simulink model "Assignment1"  (R2024a)
settings: Solver=FixedStepAuto  StartTime=0.0  StopTime=30  FixedStep=1e-3  RelTol=1e-3  EnableMultiTasking=on
undefined symbols (not defined in the file): D0, D1, D10, D11, D12, D13, D2, D3, D4, D5, D6, D7, D8, D9, PTA0, PTA1, PTA2, PTB23, PTB9, PTC16, PTC17, PTC2, PTC3, PTC4, PTD0, PTD1, PTD2, PTD3
libraries: frdmk64flib x19, dspstat3 x1
settings Model: ExtModeTrigDuration=5  Creator=raymo  LastModifiedBy=peter
settings SolverCC: AlgebraicLoopSolver=TrustRegion
settings OptimizationCC: EnhancedBackFolding=on  PassReuseOutputArgsAs=Individual arguments  ZeroExternalMemoryAtStartup=off  ZeroInternalMemoryAtStartup=off  MaxStackSize=64  OptimizeBlockOrder=speed  DifferentSizesBufferReuse=on  OptimizationCustomize=off  EfficientTunableParamExpr=on
settings DebuggingCC: ParameterTunabilityLossMsg=error  UnconnectedInputMsg=warning  UnconnectedOutputMsg=warning  UnconnectedLineMsg=warning
settings HardwareCC: ProdBitPerPointer=32  ProdBitPerSizeT=32  ProdBitPerPtrDiffT=32  ProdLargestAtomicInteger=Long  ProdLargestAtomicFloat=Double  ProdWordSize=32  ProdHWDeviceType=ARM Compatible->ARM Cortex
settings ModelReferenceCC: EnableRefExpFcnMdlSchedulingChecks=on
settings SFSimCC: MATLABDynamicMemAlloc=off
settings RTWCC: Description=Embedded Coder  SystemTargetFile=ert.tlc  HardwareBoard=NXP FRDM-K64F  TLCOptions="-aInlineSetEventsForThisBaseRateFcn=TLC_FALSE -aSuppressMultiTaskScheduler=TLC_FALSE  -aRateBasedStepFcn=0"  TemplateMakefile=ert_default_tmf  Toolchain=GNU Tools for ARM Embedded Processors  GPUComputeCapability=3.5
settings CodeAppCC: ForceParamTrailComments=on  IgnoreCustomStorageClasses=off  OperatorAnnotations=on  SimulinkDataObjDesc=on  SFDataObjDesc=on  InsertBlockDesc=on

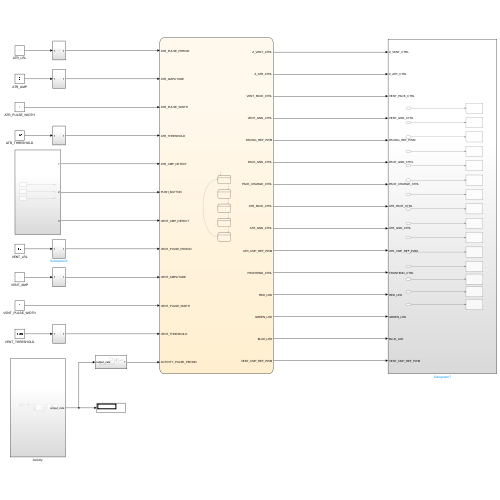
[thumbnail: Simulink's stored preview of the top-level diagram]
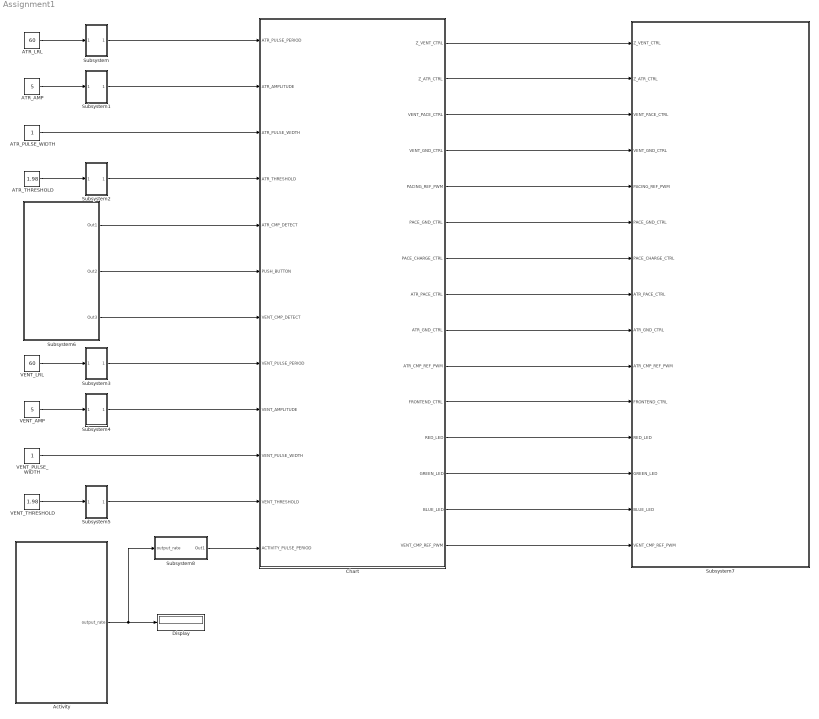
== system Assignment1 ==
  ATR_AMP : Constant  Value=5
  ATR_LRL : Constant  Value=60
  ATR_PULSE_WIDTH : Constant
  ATR_THRESHOLD : Constant  Value=1.98
  Activity : Subsystem
  Chart : Stateflow chart  TreatAsAtomicUnit=on
      settings: PortSchema="{\"entries\":[{\"content\":{\"sides\":[{\"content\":{\"connectorIds\":[\"In1\",\"In2\",\"In3\",\"In4\",\"In5\",\"In6\",\"In9\",\"In7\",\"In8\",\"In10\",\"In11\",\"In12\"]},\"type\":\"ConnectorPlacement.EquallySpacedRectSide\",\"uuid\":\"1d074b9c-7cc8-4198-85a6-5618993573f0\"},{\"content\":{\"connectorIds\":[\"Out1\",\"Out2\",\"Out3\",\"Out4\",\"Out5\",\"Out6\",\"Out7\",\"Out8\",\"Out9\",\"Out10\",\"Out11\",\"Out12\",\"Out13\",\"Out14\",\"Out15\"],\"side\":\"RIGHT\"},\"type\":\"ConnectorPlacement.EquallySpacedRectSide\",\"uuid\":\"14c2042e-8be8-4cb1-bcfb-7c1019a33e21\"},{\"content\":{\"side\":\"TOP\"},\"type\":\"ConnectorPlacement.EquallySpacedRectSide\",\"uuid\":\"e4fcd7b9-cecf-490a-a51f-afb907c3ace7\"}]},\"type\":\"ConnectorPlacement.EquallySpacedConnector\",\"uuid\":\"e4f7c1e4-ab35-4f24-879f-75d9e4e0e882\"}],\"packageUris\":[\"http://schema.mathworks.com/mf0/Connector/R2020b\"],\"version\":\"1.0\"}"
  Display : Display
  Subsystem : Subsystem
  Subsystem1 : Subsystem
  Subsystem2 : Subsystem
  Subsystem3 : Subsystem
  Subsystem4 : Subsystem
  Subsystem5 : Subsystem
  Subsystem6 : Subsystem
  Subsystem7 : Subsystem
  Subsystem8 : Subsystem
  VENT_AMP : Constant  Value=5
  VENT_LRL : Constant  Value=60
  VENT_PULSE_WIDTH : Constant
  VENT_THRESHOLD : Constant  Value=1.98
  wires:
  ATR_PULSE_WIDTH/1 -> Chart/3(ATR_PULSE_WIDTH)
  ATR_LRL/1 -> Subsystem/1(In1)
  Subsystem/1(Out1) -> Chart/1(ATR_PULSE_PERIOD)
  ATR_AMP/1 -> Subsystem1/1(In1)
  Subsystem1/1(Out1) -> Chart/2(ATR_AMPLITUDE)
  ATR_THRESHOLD/1 -> Subsystem2/1(In1)
  Subsystem2/1(Out1) -> Chart/4(ATR_THRESHOLD)
  Subsystem3/1(Out1) -> Chart/7(VENT_PULSE_PERIOD)
  VENT_LRL/1 -> Subsystem3/1(In1)
  VENT_AMP/1 -> Subsystem4/1(In1)
  Subsystem4/1(Out1) -> Chart/8(VENT_AMPLITUDE)
  VENT_PULSE_WIDTH/1 -> Chart/10(VENT_PULSE_WIDTH)
  VENT_THRESHOLD/1 -> Subsystem5/1(In1)
  Subsystem5/1(Out1) -> Chart/11(VENT_THRESHOLD)
  Subsystem6/1(Out1) -> Chart/5(ATR_CMP_DETECT)
  Subsystem6/2(Out2) -> Chart/6(PUSH_BUTTON)
  Subsystem6/3(Out3) -> Chart/9(VENT_CMP_DETECT)
  Chart/1(Z_VENT_CTRL) -> Subsystem7/1(Z_VENT_CTRL)
  Chart/2(Z_ATR_CTRL) -> Subsystem7/2(Z_ATR_CTRL)
  Chart/3(VENT_PACE_CTRL) -> Subsystem7/3(VENT_PACE_CTRL)
  Chart/4(VENT_GND_CTRL) -> Subsystem7/4(VENT_GND_CTRL)
  Chart/5(PACING_REF_PWM) -> Subsystem7/5(PACING_REF_PWM)
  Chart/6(PACE_GND_CTRL) -> Subsystem7/6(PACE_GND_CTRL)
  Chart/7(PACE_CHARGE_CTRL) -> Subsystem7/7(PACE_CHARGE_CTRL)
  Chart/8(ATR_PACE_CTRL) -> Subsystem7/8(ATR_PACE_CTRL)
  Chart/9(ATR_GND_CTRL) -> Subsystem7/9(ATR_GND_CTRL)
  Chart/10(ATR_CMP_REF_PWM) -> Subsystem7/10(ATR_CMP_REF_PWM)
  Chart/11(FRONTEND_CTRL) -> Subsystem7/11(FRONTEND_CTRL)
  Chart/12(RED_LED) -> Subsystem7/12(RED_LED)
  Chart/13(GREEN_LED) -> Subsystem7/13(GREEN_LED)
  Chart/15(VENT_CMP_REF_PWM) -> Subsystem7/15(VENT_CMP_REF_PWM)
  Activity/1(output_rate) -> Display/1, Subsystem8/1(output_rate)
  Subsystem8/1(Out1) -> Chart/12(ACTIVITY_PULSE_PERIOD)
  Chart/14(BLUE_LED) -> Subsystem7/14(BLUE_LED)

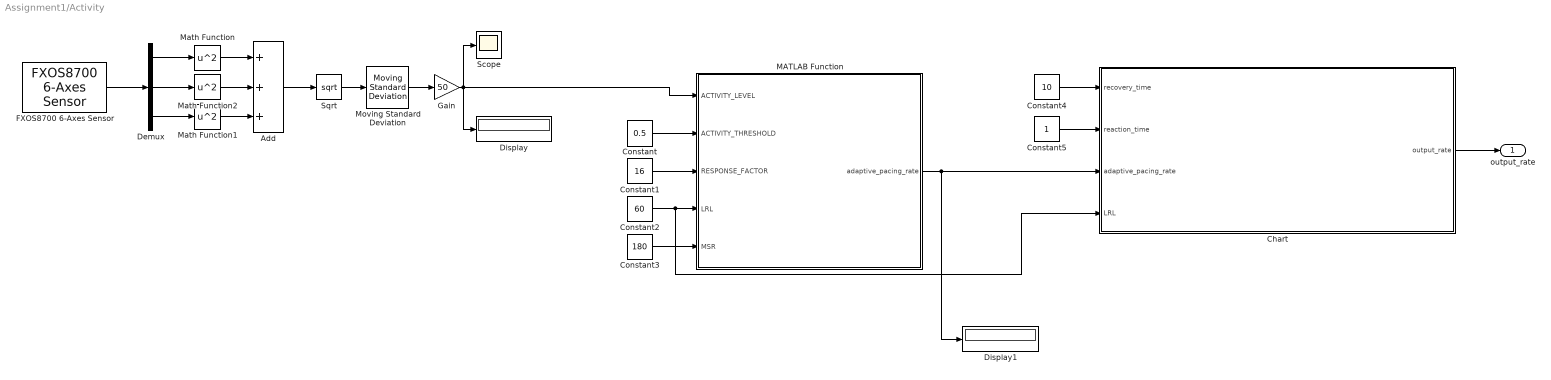
== system Assignment1/Activity ==
  Add : Sum  Inputs=+++
  Chart : Stateflow chart  TreatAsAtomicUnit=on
  Constant : Constant  Value=0.5
  Constant1 : Constant  Value=16
  Constant2 : Constant  Value=60
  Constant3 : Constant  Value=180
  Constant4 : Constant  Value=10
  Constant5 : Constant
  Demux : Demux  Outputs=3
  Display : Display
  Display1 : Display
  FXOS8700 6-Axes Sensor : frdmk64flib/FXOS8700 6-Axes Sensor  Activesensor=Accelerometer only  ODR=800Hz  HybridODR=400Hz  Accelfullrange=-4g to +4g  SampleTime=-1
  Gain : Gain  Gain=50
  MATLAB Function : MATLAB Function  TreatAsAtomicUnit=on
  Math Function : Math  Operator=square
  Math Function1 : Math  Operator=square
  Math Function2 : Math  Operator=square
  Moving Standard Deviation : dspstat3/Moving Standard Deviation  Method=Sliding window  ForgettingFactorPort=off  SpecifyWindowLength=on  WindowLength=4  OverlapLength=3  AllowArbitraryInputLength=off  ForgettingFactor=0.9  SimulateUsing=Interpreted execution
  Scope : Scope
  Sqrt : Sqrt
  output_rate : Outport
  wires:
  FXOS8700 6-Axes Sensor/1 -> Demux/1
  Demux/3 -> Math Function1/1
  Demux/2 -> Math Function2/1
  Demux/1 -> Math Function/1
  Math Function/1 -> Add/1
  Math Function2/1 -> Add/2
  Math Function1/1 -> Add/3
  Add/1 -> Sqrt/1
  Sqrt/1 -> Moving Standard Deviation/1
  Moving Standard Deviation/1 -> Gain/1
  Gain/1 -> Display/1, MATLAB Function/1(ACTIVITY_LEVEL), Scope/1
  Constant/1 -> MATLAB Function/2(ACTIVITY_THRESHOLD)
  Constant1/1 -> MATLAB Function/3(RESPONSE_FACTOR)
  Constant2/1 -> Chart/4(LRL), MATLAB Function/4(LRL)
  Constant3/1 -> MATLAB Function/5(MSR)
  MATLAB Function/1(adaptive_pacing_rate) -> Display1/1, Chart/3(adaptive_pacing_rate)
  Constant4/1 -> Chart/1(recovery_time)
  Constant5/1 -> Chart/2(reaction_time)
  Chart/1(output_rate) -> output_rate/1

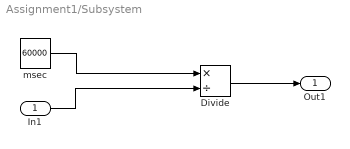
== system Assignment1/Subsystem ==
  In1 : Inport
  Divide : Product  Inputs=*/
  msec : Constant  Value=60000
  Out1 : Outport
  wires:
  Divide/1 -> Out1/1
  msec/1 -> Divide/1
  In1/1 -> Divide/2

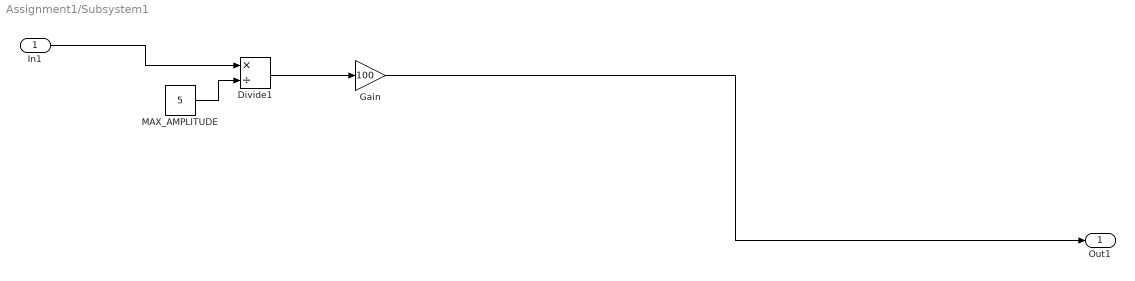
== system Assignment1/Subsystem1 ==
  In1 : Inport
  Divide1 : Product  Inputs=*/
  Gain : Gain  Gain=100
  MAX_AMPLITUDE : Constant  Value=5
  Out1 : Outport
  wires:
  Gain/1 -> Out1/1
  MAX_AMPLITUDE/1 -> Divide1/2
  In1/1 -> Divide1/1
  Divide1/1 -> Gain/1

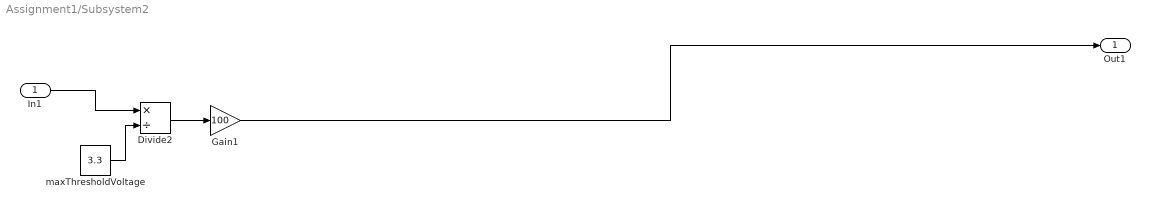
== system Assignment1/Subsystem2 ==
  In1 : Inport
  Divide2 : Product  Inputs=*/
  Gain1 : Gain  Gain=100
  maxThresholdVoltage : Constant  Value=3.3
  Out1 : Outport
  wires:
  Divide2/1 -> Gain1/1
  maxThresholdVoltage/1 -> Divide2/2
  In1/1 -> Divide2/1
  Gain1/1 -> Out1/1

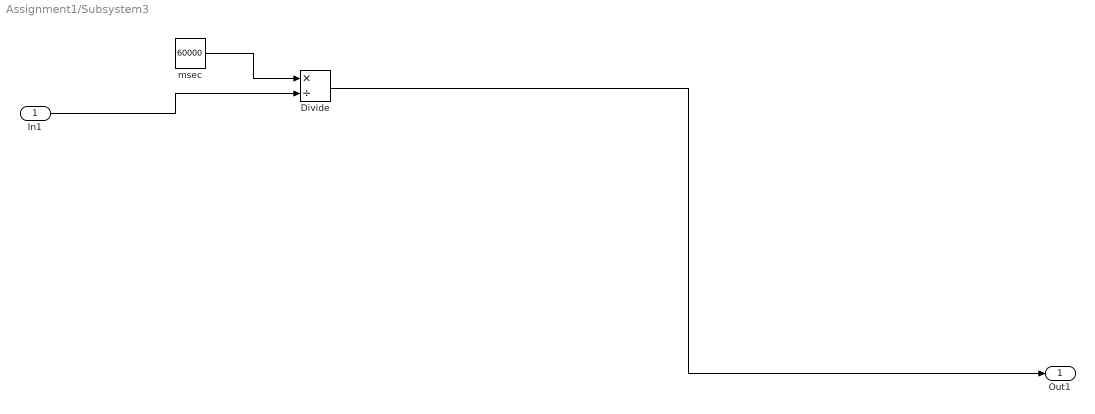
== system Assignment1/Subsystem3 ==
  In1 : Inport
  Divide : Product  Inputs=*/
  msec : Constant  Value=60000
  Out1 : Outport
  wires:
  Divide/1 -> Out1/1
  msec/1 -> Divide/1
  In1/1 -> Divide/2

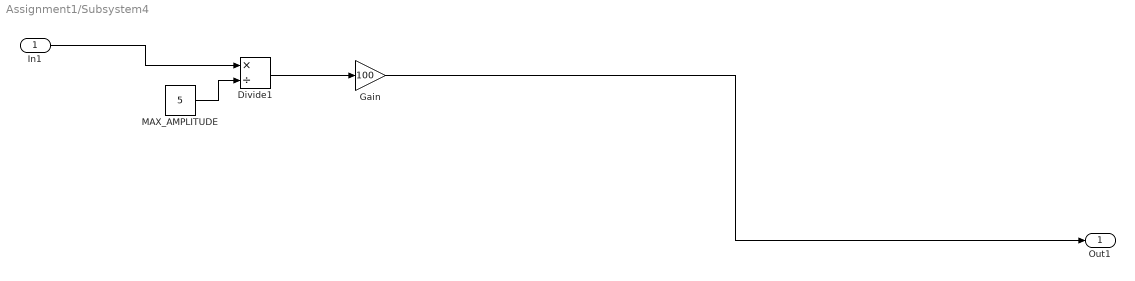
== system Assignment1/Subsystem4 ==
  In1 : Inport
  Divide1 : Product  Inputs=*/
  Gain : Gain  Gain=100
  MAX_AMPLITUDE : Constant  Value=5
  Out1 : Outport
  wires:
  Gain/1 -> Out1/1
  MAX_AMPLITUDE/1 -> Divide1/2
  In1/1 -> Divide1/1
  Divide1/1 -> Gain/1

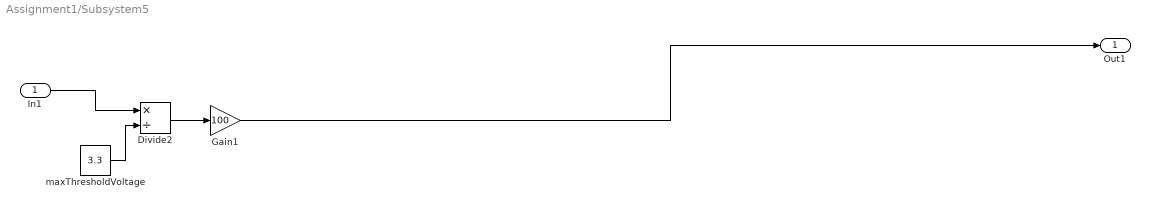
== system Assignment1/Subsystem5 ==
  In1 : Inport
  Divide2 : Product  Inputs=*/
  Gain1 : Gain  Gain=100
  maxThresholdVoltage : Constant  Value=3.3
  Out1 : Outport
  wires:
  Divide2/1 -> Gain1/1
  maxThresholdVoltage/1 -> Divide2/2
  In1/1 -> Divide2/1
  Gain1/1 -> Out1/1

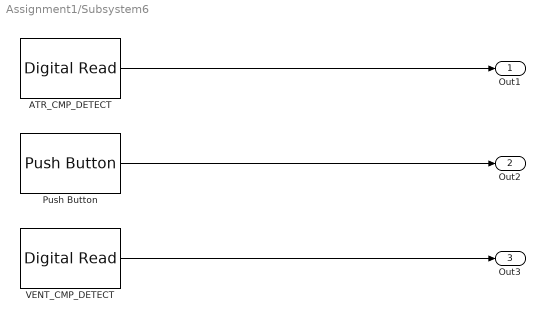
== system Assignment1/Subsystem6 ==
  ATR_CMP_DETECT : frdmk64flib/Digital Read  Whichpin=PTC16 (D0)  SampleTime=-1
  Push Button : frdmk64flib/Push Button  Whichswitch=SW2  SampleTime1=-1
  VENT_CMP_DETECT : frdmk64flib/Digital Read  Whichpin=PTC17 (D1)  SampleTime=-1
  Out1 : Outport
  Out2 : Outport  Port=2
  Out3 : Outport  Port=3
  wires:
  VENT_CMP_DETECT/1 -> Out3/1
  ATR_CMP_DETECT/1 -> Out1/1
  Push Button/1 -> Out2/1

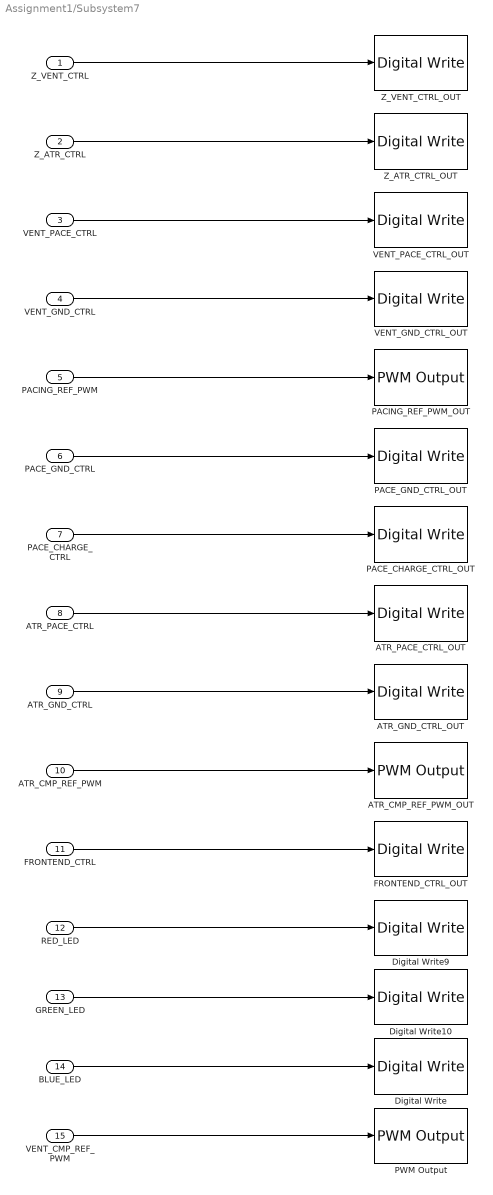
== system Assignment1/Subsystem7 ==
  Z_VENT_CTRL : Inport
  Z_ATR_CTRL : Inport  Port=2
  VENT_PACE_CTRL : Inport  Port=3
  VENT_GND_CTRL : Inport  Port=4
  PACING_REF_PWM : Inport  Port=5
  PACE_GND_CTRL : Inport  Port=6
  PACE_CHARGE_CTRL : Inport  Port=7
  ATR_PACE_CTRL : Inport  Port=8
  ATR_GND_CTRL : Inport  Port=9
  ATR_CMP_REF_PWM : Inport  Port=10
  FRONTEND_CTRL : Inport  Port=11
  RED_LED : Inport  Port=12
  GREEN_LED : Inport  Port=13
  BLUE_LED : Inport  Port=14
  VENT_CMP_REF_PWM : Inport  Port=15
  ATR_CMP_REF_PWM_OUT : frdmk64flib/PWM Output  Whichpin=PTC2 (D6)  InitialFrequency=2000  InitialDutyCycle=50
  ATR_GND_CTRL_OUT : frdmk64flib/Digital Write  Whichpin=PTD2 (D11)
  ATR_PACE_CTRL_OUT : frdmk64flib/Digital Write  Whichpin=PTA0 (D8)
  Digital Write : frdmk64flib/Digital Write  Whichpin=BLUE_LED
  Digital Write10 : frdmk64flib/Digital Write  Whichpin=GREEN_LED
  Digital Write9 : frdmk64flib/Digital Write  Whichpin=RED_LED
  FRONTEND_CTRL_OUT : frdmk64flib/Digital Write  Whichpin=PTD1 (D13)
  PACE_CHARGE_CTRL_OUT : frdmk64flib/Digital Write  Whichpin=PTB9 (D2)
  PACE_GND_CTRL_OUT : frdmk64flib/Digital Write  Whichpin=PTD0 (D10)
  PACING_REF_PWM_OUT : frdmk64flib/PWM Output  Whichpin=PTA2 (D5)  InitialFrequency=2000  InitialDutyCycle=50
  PWM Output : frdmk64flib/PWM Output  Whichpin=PTA1 (D3)  InitialFrequency=2000  InitialDutyCycle=0
  VENT_GND_CTRL_OUT : frdmk64flib/Digital Write  Whichpin=PTD3 (D12)
  VENT_PACE_CTRL_OUT : frdmk64flib/Digital Write  Whichpin=PTC4 (D9)
  Z_ATR_CTRL_OUT : frdmk64flib/Digital Write  Whichpin=PTB23 (D4)
  Z_VENT_CTRL_OUT : frdmk64flib/Digital Write  Whichpin=PTC3 (D7)
  wires:
  ATR_PACE_CTRL/1 -> ATR_PACE_CTRL_OUT/1
  PACE_GND_CTRL/1 -> PACE_GND_CTRL_OUT/1
  Z_VENT_CTRL/1 -> Z_VENT_CTRL_OUT/1
  PACE_CHARGE_CTRL/1 -> PACE_CHARGE_CTRL_OUT/1
  GREEN_LED/1 -> Digital Write10/1
  ATR_CMP_REF_PWM/1 -> ATR_CMP_REF_PWM_OUT/1
  RED_LED/1 -> Digital Write9/1
  ATR_GND_CTRL/1 -> ATR_GND_CTRL_OUT/1
  FRONTEND_CTRL/1 -> FRONTEND_CTRL_OUT/1
  VENT_GND_CTRL/1 -> VENT_GND_CTRL_OUT/1
  PACING_REF_PWM/1 -> PACING_REF_PWM_OUT/1
  VENT_PACE_CTRL/1 -> VENT_PACE_CTRL_OUT/1
  Z_ATR_CTRL/1 -> Z_ATR_CTRL_OUT/1
  VENT_CMP_REF_PWM/1 -> PWM Output/1
  BLUE_LED/1 -> Digital Write/1

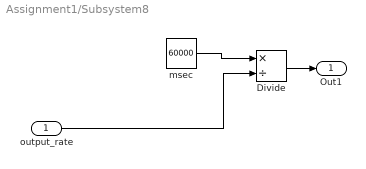
== system Assignment1/Subsystem8 ==
  output_rate : Inport
  Divide : Product  Inputs=*/
  msec : Constant  Value=60000
  Out1 : Outport
  wires:
  output_rate/1 -> Divide/2
  msec/1 -> Divide/1
  Divide/1 -> Out1/1

== stateflow chart Assignment1/Activity/Chart ==
  state IDLE
    entry:
    output_rate = LRL;
  state INIT
    entry:
    %The slope of the time response curves
    step_up = abs((adaptive_pacing_rate - output_rate)/reaction_time);
    step_down = abs((adaptive_pacing_rate - output_rate)/recovery_time);
  state STEP_DOWN
    entry:
    output_rate = output_rate - step_down;
  state STEP_UP
    entry:
    output_rate = output_rate + step_up;
  (default) -> IDLE
  IDLE -> INIT
  INIT -> STEP_DOWN [order 2] : [output_rate > adaptive_pacing_rate]
  INIT -> STEP_UP [order 1] : [output_rate < adaptive_pacing_rate]
  STEP_UP -> INIT : [after(1000,msec)]
  STEP_DOWN -> INIT : [after(1000,msec)]
  data: recovery_time input; reaction_time input; adaptive_pacing_rate input; LRL input; step_down local; step_up local; output_rate output

== matlab function Assignment1/Activity/MATLAB Function ==
  data: ACTIVITY_LEVEL input; adaptive_pacing_rate output; ACTIVITY_THRESHOLD input; RESPONSE_FACTOR input; LRL input; MSR input
function adaptive_pacing_rate = fcn(ACTIVITY_LEVEL, ACTIVITY_THRESHOLD, RESPONSE_FACTOR, LRL , MSR)
    if ACTIVITY_LEVEL <= ACTIVITY_THRESHOLD
        adaptive_pacing_rate = LRL; 
    else
        slope = 2.5*RESPONSE_FACTOR;
        b = LRL - (slope*ACTIVITY_THRESHOLD);
        linear_rate_response = (slope*ACTIVITY_LEVEL) + b;
        if(linear_rate_response >= MSR)
           adaptive_pacing_rate = MSR;
        else
            adaptive_pacing_rate = linear_rate_response;
        end
    end
end

== stateflow chart Assignment1/Chart ==
  state AOO
    state ChargeDishcharge
      entry:
      %C22
      ATR_PACE_CTRL = 0;
      VENT_PACE_CTRL = 0;
      PACING_REF_PWM = ATR_AMPLITUDE;
      PACE_CHARGE_CTRL = 1;
      %C21
      PACE_GND_CTRL = 1;
      VENT_PACE_CTRL = 0;
      Z_ATR_CTRL = 0;
      Z_VENT_CTRL = 0;
      ATR_GND_CTRL = 1;
      VENT_GND_CTRL = 0;
      %LED
      RED_LED = 0;
      GREEN_LED = 0;
      BLUE_LED = 0;
    state AVpacing
      entry:
      PACE_CHARGE_CTRL = 0;
      PACE_GND_CTRL = 1;
      ATR_PACE_CTRL = 1;
      ATR_GND_CTRL = 0;
      Z_ATR_CTRL = 0;
      Z_VENT_CTRL = 0;
      VENT_GND_CTRL = 0;
      VENT_PACE_CTRL = 0;
      PACING_REF_PWM = ATR_AMPLITUDE;
    (default) -> AOO.ChargeDishcharge
    AOO.AVpacing -> AOO.ChargeDishcharge : [after(ATR_PULSE_WIDTH, msec)]
    AOO.ChargeDishcharge -> AOO.AVpacing : [after(ATR_PULSE_PERIOD-ATR_PULSE_WIDTH, msec)]
  state AAI
    state Idle
      entry:
      %Set threshold
      ATR_CMP_REF_PWM = ATR_THRESHOLD;
      FRONTEND_CTRL = 1;
      RED_LED = 1;
      GREEN_LED = 0;
      BLUE_LED = 0;
    state AVpacing
      entry:
      PACE_CHARGE_CTRL = 0;
      PACE_GND_CTRL = 1;
      ATR_PACE_CTRL = 1;
      ATR_GND_CTRL = 0;
      Z_ATR_CTRL = 0;
      Z_VENT_CTRL = 0;
      VENT_GND_CTRL = 0;
      VENT_PACE_CTRL = 0;
      PACING_REF_PWM = ATR_AMPLITUDE;
    state ChargeDischarge
      entry:
      %C22
      ATR_PACE_CTRL = 0;
      VENT_PACE_CTRL = 0;
      PACING_REF_PWM = ATR_AMPLITUDE;
      PACE_CHARGE_CTRL = 1;
      %C21
      PACE_GND_CTRL = 1;
      VENT_PACE_CTRL = 0;
      Z_ATR_CTRL = 0;
      Z_VENT_CTRL = 0;
      ATR_GND_CTRL = 1;
      VENT_GND_CTRL = 0;
    (default) -> Idle
    Idle -> ChargeDischarge
    ChargeDischarge -> ChargeDischarge [order 1] : after(5,msec)[ATR_CMP_DETECT == 1]
    ChargeDischarge -> AAI.AVpacing [order 2] : [after(ATR_PULSE_PERIOD-ATR_PULSE_WIDTH,msec)]
    AAI.AVpacing -> ChargeDischarge : [after(ATR_PULSE_WIDTH, msec)]
  state VOO
    state Pacing
      entry:
      PACE_CHARGE_CTRL=0;
      PACE_GND_CTRL=1;
      ATR_PACE_CTRL=0;
      ATR_GND_CTRL=0;
      Z_ATR_CTRL=0;
      Z_VENT_CTRL=0;
      VENT_GND_CTRL=0;
      VENT_PACE_CTRL=1;
    state Charging
      entry:
      ATR_PACE_CTRL=0;
      VENT_PACE_CTRL=0;
      PACING_REF_PWM=VENT_AMPLITUDE;
      PACE_CHARGE_CTRL=1;
      RED_LED = 0;
      GREEN_LED = 1;
      BLUE_LED = 0;
    state Discharging
      entry:
      PACE_GND_CTRL=1;
      VENT_PACE_CTRL=0;
      Z_ATR_CTRL=0;
      Z_VENT_CTRL=0;
      ATR_PACE_CTRL=0;
      ATR_GND_CTRL=0;
      VENT_GND_CTRL=1;
    (default) -> VOO.Charging
    VOO.Charging -> VOO.Pacing : [after(VENT_PULSE_PERIOD,msec)]
    VOO.Discharging -> VOO.Charging
    VOO.Pacing -> VOO.Discharging : [after(VENT_PULSE_WIDTH,msec)]
  state VVI
    state Initialization
      entry:
      FRONTEND_CTRL = 1;
      VENT_CMP_REF_PWM = VENT_THRESHOLD;
      RED_LED = 1;
      GREEN_LED = 1;
      BLUE_LED = 0;
    state Pacing
      entry:
      PACE_CHARGE_CTRL=0;
      PACE_GND_CTRL=1;
      ATR_PACE_CTRL=0;
      ATR_GND_CTRL=0;
      Z_ATR_CTRL=0;
      Z_VENT_CTRL=0;
      VENT_GND_CTRL=0;
      VENT_PACE_CTRL=1;
    state Charging
      entry:
      ATR_PACE_CTRL=0;
      VENT_PACE_CTRL=0;
      PACING_REF_PWM=VENT_AMPLITUDE;
      PACE_CHARGE_CTRL=1;
    state Discharging
      entry:
      PACE_GND_CTRL=1;
      VENT_PACE_CTRL=0;
      Z_ATR_CTRL=0;
      Z_VENT_CTRL=0;
      ATR_PACE_CTRL=0;
      ATR_GND_CTRL=0;
      VENT_GND_CTRL=1;
    (default) -> Initialization
    VVI.Charging -> VVI.Charging [order 1] : after(5,msec)[VENT_CMP_DETECT == 1]
    Initialization -> VVI.Charging
    VVI.Charging -> VVI.Pacing [order 2] : [after(VENT_PULSE_PERIOD-VENT_PULSE_WIDTH,msec)]
    VVI.Discharging -> VVI.Charging
    VVI.Pacing -> VVI.Discharging : [after(VENT_PULSE_WIDTH,msec)]
  state AOOR
    state ChargeDishcharge
      entry:
      %C22
      ATR_PACE_CTRL = 0;
      VENT_PACE_CTRL = 0;
      PACING_REF_PWM = ATR_AMPLITUDE;
      PACE_CHARGE_CTRL = 1;
      %C21
      PACE_GND_CTRL = 1;
      VENT_PACE_CTRL = 0;
      Z_ATR_CTRL = 0;
      Z_VENT_CTRL = 0;
      ATR_GND_CTRL = 1;
      VENT_GND_CTRL = 0;
      %LED
      RED_LED = 0;
      GREEN_LED = 0;
      BLUE_LED = 1;
    state AVpacing
      entry:
      PACE_CHARGE_CTRL = 0;
      PACE_GND_CTRL = 1;
      ATR_PACE_CTRL = 1;
      ATR_GND_CTRL = 0;
      Z_ATR_CTRL = 0;
      Z_VENT_CTRL = 0;
      VENT_GND_CTRL = 0;
      VENT_PACE_CTRL = 0;
      PACING_REF_PWM = ATR_AMPLITUDE;
    (default) -> AOOR.ChargeDishcharge
    AOOR.AVpacing -> AOOR.ChargeDishcharge : [after(ATR_PULSE_WIDTH, msec)]
    AOOR.ChargeDishcharge -> AOOR.AVpacing : [after(ACTIVITY_PULSE_PERIOD-ATR_PULSE_WIDTH, msec)]
  state VOOR
    state Pacing
      entry:
      PACE_CHARGE_CTRL=0;
      PACE_GND_CTRL=1;
      ATR_PACE_CTRL=0;
      ATR_GND_CTRL=0;
      Z_ATR_CTRL=0;
      Z_VENT_CTRL=0;
      VENT_GND_CTRL=0;
      VENT_PACE_CTRL=1;
    state Charging
      entry:
      ATR_PACE_CTRL=0;
      VENT_PACE_CTRL=0;
      PACING_REF_PWM=VENT_AMPLITUDE;
      PACE_CHARGE_CTRL=1;
      RED_LED = 1;
      GREEN_LED = 0;
      BLUE_LED = 1;
    state Discharging
      entry:
      PACE_GND_CTRL=1;
      VENT_PACE_CTRL=0;
      Z_ATR_CTRL=0;
      Z_VENT_CTRL=0;
      ATR_PACE_CTRL=0;
      ATR_GND_CTRL=0;
      VENT_GND_CTRL=1;
    (default) -> VOOR.Charging
    VOOR.Charging -> VOOR.Pacing : [after(ACTIVITY_PULSE_PERIOD,msec)]
    VOOR.Discharging -> VOOR.Charging
    VOOR.Pacing -> VOOR.Discharging : [after(VENT_PULSE_WIDTH,msec)]
  (default) -> AOO
  VOOR -> AOO : after(500,msec)[PUSH_BUTTON == 1]
  AOO -> AAI : after(500,msec)[PUSH_BUTTON == 1]
  AAI -> VOO : after(500,msec)[PUSH_BUTTON == 1]
  VOO -> VVI : after(500,msec)[PUSH_BUTTON == 1]
  VVI -> AOOR : after(500,msec)[PUSH_BUTTON == 1]
  AOOR -> VOOR : after(500,msec)[PUSH_BUTTON == 1]
  data: ATR_PULSE_PERIOD input; ATR_AMPLITUDE input; ATR_PULSE_WIDTH input; ATR_THRESHOLD input; ATR_CMP_DETECT input; Z_VENT_CTRL output; Z_ATR_CTRL output; VENT_PACE_CTRL output; VENT_GND_CTRL output; PACING_REF_PWM output; PACE_GND_CTRL output; PACE_CHARGE_CTRL output; ATR_PACE_CTRL output; ATR_GND_CTRL output; ATR_CMP_REF_PWM output; FRONTEND_CTRL output; PUSH_BUTTON input; RED_LED output; GREEN_LED output; BLUE_LED output; VENT_PULSE_PERIOD input; VENT_CMP_REF_PWM output; VENT_AMPLITUDE input; VENT_CMP_DETECT input; VENT_PULSE_WIDTH input; VENT_THRESHOLD input; ACTIVITY_PULSE_PERIOD input
